simulink model "renovables"  (R2018a)
settings: Solver=ode8  StartTime=0.0  StopTime=10.0  FixedStep=0.0001  RelTol=1e-3
InitFcn:
  | SimulinkInit_linea_transmision
values from neighbouring files (symbols this model uses):
  C2 = 22e-6    (= 2.2e-05)    [SimulinkInit_linea_transmision.m]
  L2 = 30e-3    (= 0.03)    [SimulinkInit_linea_transmision.m]
  L5 = 22e-6    (= 2.2e-05)    [SimulinkInit_linea_transmision.m]
  R2 = 0.2    [SimulinkInit_linea_transmision.m]
  R5 = 0.0012    [SimulinkInit_linea_transmision.m]
libraries: dsparch4 x2, powerlib_meascontrol x1
settings Model: Creator=MarioAndres  LastModifiedBy=MarioAndres
settings OptimizationCC: DefaultParameterBehavior=Inlined  EnhancedBackFolding=on  PassReuseOutputArgsAs=Individual arguments  OptimizeBlockOrder=speed  DifferentSizesBufferReuse=on  OptimizationCustomize=off
settings DebuggingCC: ParameterTunabilityLossMsg=error
settings SFSimCC: MATLABDynamicMemAlloc=off
settings RTWCC: SystemTargetFile=ert.tlc  TemplateMakefile=ert_default_tmf  GenerateReport=on  IncludeHyperlinkInReport=on  LaunchReport=on  GenerateTraceInfo=on  GenerateTraceReport=on  GenerateTraceReportSl=on  GenerateTraceReportSf=on  GenerateTraceReportEml=on
settings CodeAppCC: ForceParamTrailComments=on  IgnoreCustomStorageClasses=off  OperatorAnnotations=on  SimulinkDataObjDesc=on  SFDataObjDesc=on  InsertBlockDesc=on
settings ERTTargetCC: TargetLangStandard=C99 (ISO)  GenerateSampleERTMain=on  SupportContinuousTime=on  InlinedParameterPlacement=NonHierarchical  ERTCustomFileTemplate=example_file_process.tlc

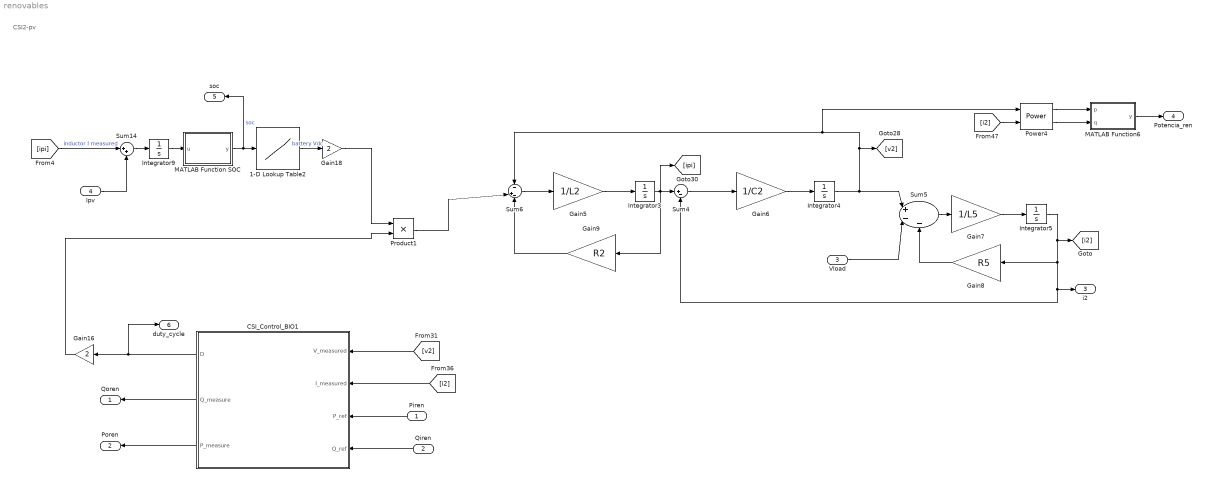
== system renovables ==
  note: CSI2-pv
  Piren : Inport
  Qiren : Inport  Port=2
  Vload : Inport  Port=3
  Ipv : Inport  Port=4
  1-D Lookup Table2 : Lookup_n-D  NumberOfTableDimensions=1  BreakpointsForDimension1=[0 10 20 30 40 50 70 80 100]  Table=[0 10 200 500 800 1000 1140 1150 1200]  InternalRulePriority=Speed  RndMeth=Simplest  InputSameDT=on
  CSI_Control_BIO1 : Subsystem  mask{A=[0.0201   -0.039932     0.01986], B=[1     -1.9966       0.998], T=0.0001, st_time=.1, Dn=[1     -1.0364], Dd=[1    -0.96364]}
      mask prompts: A "Numerador del control PR(z)"; B "Denominador del control PR(z)"; T "Tiempo de muestreo"; st_time "Tiempo_muerto"; Dn "Dn (Numerador de D(z))"; Dd "Dd (numerador de D(z))"
      mask DialogControl descripcion Prompt: Lazo de control de corriente para inversor monofasico. La entrada es un setpoint de potencia [P, Q]. Con ese setpoint se calcula la referencia de corriente sinusoidal deacuerdo a la tension medida de la red. Por lo anterior este controlador solo es valido para un inversor conectado a la red pues hara que se comporte como un CSI.
      mask DialogControl Control2 Prompt: Dn y Dd corresponden al numerador y denominador de la funcion de transferencia en Z (denominada D(z)) que hara un desfase de 90 de las señales medidas de tension y corriente del inversor. Estos desfases permiten mimificar las señales alfa y beta, de esta forma usar la misma teoria de potencia instantanea para el caso monofasico.
  Gain16 : Gain  Gain=2
  Gain18 : Gain  Gain=2
  Gain5 : Gain  Gain=1/L2
  Gain6 : Gain  Gain=1/C2
  Gain7 : Gain  Gain=1/L5
  Gain8 : Gain  Gain=R5
  Gain9 : Gain  Gain=R2
  Integrator3 : Integrator
  Integrator4 : Integrator
  Integrator5 : Integrator
  Integrator9 : Integrator  LimitOutput=on  UpperSaturationLimit=1  LowerSaturationLimit=0
  "MATLAB Function SOC " : MATLAB Function  TreatAsAtomicUnit=on
  MATLAB Function6 : MATLAB Function  TreatAsAtomicUnit=on
  Power4 : powerlib_meascontrol/Measurements/Power  Freq=60  Vinit=[1, 0]  Iinit=[1, 0]  Ts=0
      settings: SourceProductName=Simscape Power Systems
  Product1 : Product
  Sum14 : Sum  Inputs=|++
  Sum4 : Sum  Inputs=|+-
  Sum5 : Sum  Inputs=|+--
  Sum6 : Sum  Inputs=-|+-
  Qoren : Outport
  Poren : Outport  Port=2
  i2 : Outport  Port=3
  Potencia_ren : Outport  Port=4
  soc : Outport  Port=5
  duty_cycle : Outport  Port=6
  wires:
  Sum5/1 -> Gain7/1
  "MATLAB Function SOC "/1(y) -> soc/1, 1-D Lookup Table2/1  "soc"
  Integrator3/1 -> [ipi], Gain9/1, Sum4/1
  1-D Lookup Table2/1 -> Gain18/1  "battery Vdc"
  Power4/1 -> MATLAB Function6/1(p)
  Integrator9/1 -> "MATLAB Function SOC "/1(u)
  [i2] -> CSI_Control_BIO1/2(I_measured)
  MATLAB Function6/1(y) -> Potencia_ren/1
  Gain7/1 -> Integrator5/1
  Gain16/1 -> Product1/2
  Gain18/1 -> Product1/1
  Sum6/1 -> Gain5/1
  [v2] -> CSI_Control_BIO1/1(V_measured)
  Gain8/1 -> Sum5/3
  Integrator4/1 -> [v2], Power4/1, Sum6/1, Sum5/1
  Gain9/1 -> Sum6/3
  Product1/1 -> Sum6/2
  Sum4/1 -> Gain6/1
  Sum14/1 -> Integrator9/1
  Gain5/1 -> Integrator3/1
  Integrator5/1 -> [i2], i2/1, Sum4/2, Gain8/1
  [ipi] -> Sum14/1  "inductor I measured"
  Power4/2 -> MATLAB Function6/2(q)
  [i2] -> Power4/2
  Gain6/1 -> Integrator4/1
  CSI_Control_BIO1/1(D) -> duty_cycle/1, Gain16/1
  Vload/1 -> Sum5/2
  CSI_Control_BIO1/2(Q_measure) -> Qoren/1
  CSI_Control_BIO1/3(P_measure) -> Poren/1
  Qiren/1 -> CSI_Control_BIO1/4(Q_ref)
  Piren/1 -> CSI_Control_BIO1/3(P_ref)
  Ipv/1 -> Sum14/2

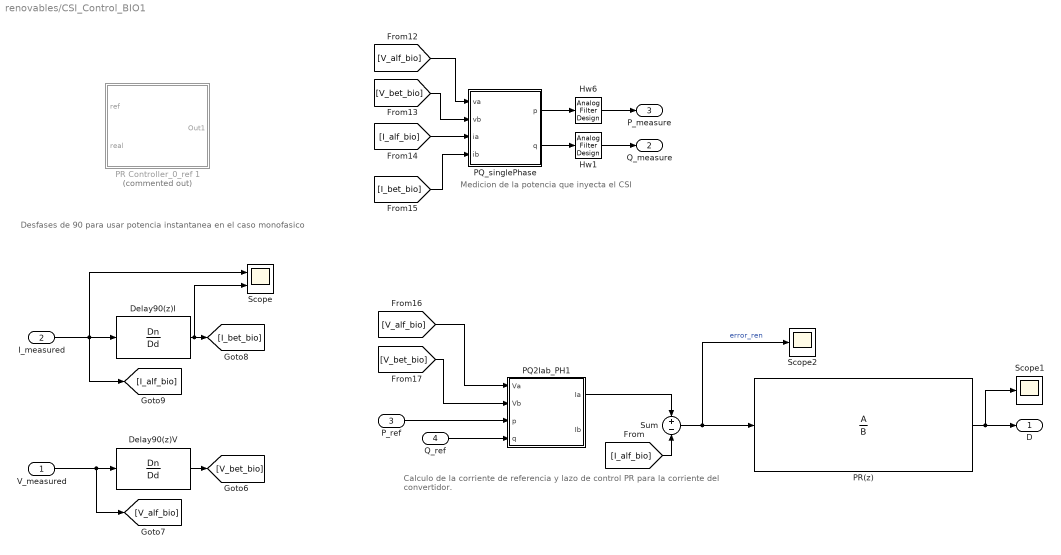
== system renovables/CSI_Control_BIO1 ==
  note: Medicion de la potencia que inyecta el CSI
  note: Desfases de 90 para usar potencia
      | instantanea en el caso monofasico
  note: Calculo de la corriente de referencia
      | y lazo de control PR para la corriente
      | del convertidor.
  V_measured : Inport
  I_measured : Inport  Port=2
  P_ref : Inport  Port=3
  Q_ref : Inport  Port=4
  Delay90(z)I : DiscreteTransferFcn  Numerator=Dn  Denominator=Dd  SampleTime=T
  Delay90(z)V : DiscreteTransferFcn  Numerator=Dn  Denominator=Dd  SampleTime=T
  Hw1 : dsparch4/Analog Filter Design  method=Bessel  filttype=Lowpass  N=4  Wlo=30*2*pi  Whi=80  Rp=2  Rs=80
  Hw6 : dsparch4/Analog Filter Design  method=Bessel  filttype=Lowpass  N=4  Wlo=30*2*pi  Whi=80  Rp=2  Rs=80
  PQ2Iab_PH1 : MATLAB Function  TreatAsAtomicUnit=on
  PQ_singlePhase : MATLAB Function  TreatAsAtomicUnit=on
  PR Controller_0_ref 1 : Subsystem  Commented=on  mask{Kp=40/100, Ki=200, wa=2, w0=60*2*pi, st_time=1e-3}
      mask prompts: Kp "Ganancia Proporcional"; Ki "Ganancia Integral"; wa "Ancho camapana resonancia"; w0 "Frecuencia Central"; st_time "Tiempo muerto (Start)"
      mask Display:
      | port_label('input',1,'ref')
      | port_label('input',2,'sens')
      | port_label('output',1,'out')
      | 
      | plot(.4+[0:.01:pi/10], .32+sin(40*[0:.01:pi/10])/13)
      | 
      | plot([.4 .6],.05+[.5 .7])
      | plot([.4 .6],.05+[.9 .7])
      | plot([.4 .4],.05+[.9 .5])
      | 
      | text(.27,.37,'\fontsize{25} \int', 'texmode', 'on')
  PR(z) : DiscreteTransferFcn  Numerator=A  Denominator=B  SampleTime=T
  Scope : Scope  NumInputPorts=2
  Scope1 : Scope
  Scope2 : Scope
  Sum : Sum  Inputs=+-
  D : Outport
  Q_measure : Outport  Port=2
  P_measure : Outport  Port=3
  wires:
  I_measured/1 -> Scope/1, Delay90(z)I/1, [I_alf_bio]
  [V_bet_bio] -> PQ2Iab_PH1/2(Vb)
  Delay90(z)I/1 -> Scope/2, [I_bet_bio]
  [I_bet_bio] -> PQ_singlePhase/4(ib)
  [I_alf_bio] -> PQ_singlePhase/3(ia)
  [V_alf_bio] -> PQ2Iab_PH1/1(Va)
  Delay90(z)V/1 -> [V_bet_bio]
  [V_bet_bio] -> PQ_singlePhase/2(vb)
  [V_alf_bio] -> PQ_singlePhase/1(va)
  V_measured/1 -> Delay90(z)V/1, [V_alf_bio]
  P_ref/1 -> PQ2Iab_PH1/3(p)
  Q_ref/1 -> PQ2Iab_PH1/4(q)
  Sum/1 -> Scope2/1, PR(z)/1  "error_ren"
  [I_alf_bio] -> Sum/2
  PQ2Iab_PH1/1(Ia) -> Sum/1
  PR(z)/1 -> Scope1/1, D/1
  PQ_singlePhase/2(q) -> Hw1/1
  Hw1/1 -> Q_measure/1
  PQ_singlePhase/1(p) -> Hw6/1
  Hw6/1 -> P_measure/1

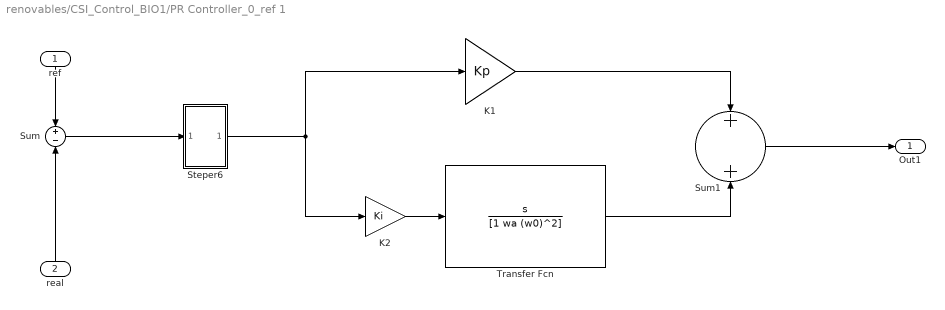
== system renovables/CSI_Control_BIO1/PR Controller_0_ref 1 ==
  ref : Inport
  real : Inport  Port=2
  K1 : Gain  Gain=Kp
  K2 : Gain  Gain=Ki
  Steper6 : Subsystem
  Sum : Sum  Inputs=+-
  Sum1 : Sum  Inputs=+|+
  Transfer Fcn : TransferFcn  Numerator=[1 0]  Denominator=[1 wa (w0)^2]
  Out1 : Outport
  wires:
  real/1 -> Sum/2
  ref/1 -> Sum/1
  Sum/1 -> Steper6/1(In1)
  K1/1 -> Sum1/1
  Transfer Fcn/1 -> Sum1/2
  K2/1 -> Transfer Fcn/1
  Steper6/1(Out1) -> K1/1, K2/1
  Sum1/1 -> Out1/1

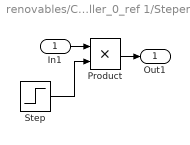
== system renovables/CSI_Control_BIO1/PR Controller_0_ref 1/Steper6 ==
  In1 : Inport
  Product : Product
  Step : Step  Time=st_time  SampleTime=0
  Out1 : Outport
  wires:
  Product/1 -> Out1/1
  In1/1 -> Product/1
  Step/1 -> Product/2

== matlab function renovables/CSI_Control_BIO1/PQ2Iab_PH1 ==
  data: Va input; Ia output; Vb input; p input; q input; Ib output
function [Ia, Ib] = fcn(Va, Vb, p, q)
%#codegen
% Ia=0;
% Ib=0;
% divide by zero protection
if(abs((Va^2+Vb^2))<=1000*eps(0))
    det = 1/eps(0);
else
    det = 1/(Va^2+Vb^2); % constante auxiliar
end
%det = 1/(Va^2+Vb^2);

Mat = det*[Va Vb; Vb -Va];

Iab = Mat*[2*p;2*q];

Iaaux = Iab(1);
Ibaux = Iab(2);

ilim=1e3;

if(Iaaux>ilim)
    Iaaux=ilim;
end
if(Iaaux<-ilim)
    Iaaux =-ilim;    
end

if(isnan(Iaaux))
    Iaaux=0;
end
%-----------------


if(Ibaux>ilim)
    Ibaux=ilim;
end
if(Ibaux<-ilim)
    Ibaux =-ilim;    
end

if(isnan(Ibaux))
    Ibaux=0;
end
%-----------------


Ia = Iaaux;
Ib = Ibaux;

== matlab function renovables/CSI_Control_BIO1/PQ_singlePhase ==
  data: va input; p output; vb input; ia input; ib input; q output
function [p, q] = fcn(va, vb, ia, ib)
% Esta funcion calcula la potencia activa y reactiva instantanea
% para el caso mnosofasico. En la revision de 2 papers he observado
% que una manera de extender la teoria de potencia al caso monofasico
% es asumiendo la tension o corriente de una fase como la componente
% alpha y hacer un desfase de 90 grados para obtener una version
% artificial de beta.

paux=va*ia+vb*ib;
if(paux > 20e4)
    paux = 20e4;
end
if(paux < -20e4)
    paux = -20e-4;
end

p = paux/2; % potencia activa instantanea

qaux = vb*ia-va*ib;

if(qaux>20e4)
    qaux=20e4;
end
if(qaux<-20e4)
    qaux=-20e4;
end

q = qaux/2; % potencia reactiva instantanea

== matlab function renovables/MATLAB Function SOC  ==
  data: u input; y output
function y = fcn(u)

y = -0.03536*u+100;

== matlab function renovables/MATLAB Function6 ==
  data: p input; y output; q input
function y = fcn(p,q)

y = sqrt(p^2+q^2);
